simulink model "PlatooningUsingV2VTestBench"  (R2025a)
settings: Solver=ode23tb  StartTime=0.0  StopTime=stopTime  RelTol=1e-1  AbsTol=5e-5
PostLoadFcn:
  | helperSLPlatooningUsingV2VSetup
InitFcn:
  | figureName = 'Platooning Simulation Results';
  | hFig = findobj('Type','Figure','Name',figureName);
  | close(hFig)
values from neighbouring files (symbols this model uses):
  L = vehicleDimension.TractorLength + vehicleDimension.TrailerLength + vehicleDimension.InterConnection - vehicleDimension.Overlap + spacing    [helperSLPlatooningUsingV2VSetup.m]
  spacing = 7    [helperSLPlatooningUsingV2VSetup.m]
undefined symbols (not defined in the file or in its folder): accelerationProfile, C1, DiscIntNeverNeededParam, initialActorPose, K1, K2, N, sceneOrigin, Sim3dSensor, tractor, Ts, Tsv, vehicleDimension
libraries: simulink x7, sim3dautolib x6, slpidlib x2, sim3dcameralib x1, sim3dlib x1, visionsinks x1
(part 2 of 2)

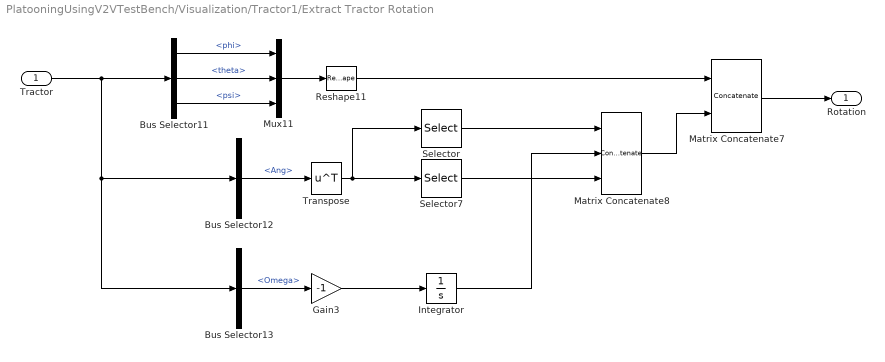
== system PlatooningUsingV2VTestBench/Visualization/Tractor1/Extract Tractor Rotation ==
  Tractor : Inport
  Bus Selector11 : BusSelector  OutputSignals=Vehicle.InertFrm.Cg.Ang.phi,Vehicle.InertFrm.Cg.Ang.theta,Vehicle.InertFrm.Cg.Ang.psi
  Bus Selector12 : BusSelector  OutputSignals=Suspension.Whl.Ang
  Bus Selector13 : BusSelector  OutputSignals=Wheels.TireFrame.Omega
  Gain3 : Gain  Gain=-1
  Integrator : Integrator
  Matrix Concatenate7 : Concatenate  Mode=Multidimensional array
  Matrix Concatenate8 : Concatenate  NumInputs=3  Mode=Multidimensional array  ConcatenateDimension=2
  Mux11 : Mux  Inputs=3
  Reshape11 : Reshape  OutputDimensionality=Row vector (2-D)
  Selector : Selector  NumberOfDimensions=2  InputPortWidth=3  IndexOptions=Select all,Index vector (dialog)  Indices=1,1  OutputSizes=1,1
  Selector7 : Selector  NumberOfDimensions=2  InputPortWidth=3  IndexOptions=Select all,Index vector (dialog)  Indices=3,3  OutputSizes=1,1
  Transpose : Math  Operator=transpose
  Rotation : Outport
  wires:
  Transpose/1 -> Selector7/1, Selector/1
  Gain3/1 -> Integrator/1
  Selector7/1 -> Matrix Concatenate8/3
  Bus Selector11/3 -> Mux11/3  "<psi>"
  Bus Selector11/1 -> Mux11/1  "<phi>"
  Bus Selector11/2 -> Mux11/2  "<theta>"
  Reshape11/1 -> Matrix Concatenate7/1
  Selector/1 -> Matrix Concatenate8/1
  Mux11/1 -> Reshape11/1
  Bus Selector12/1 -> Transpose/1  "<Ang>"
  Matrix Concatenate8/1 -> Matrix Concatenate7/2
  Tractor/1 -> Bus Selector13/1, Bus Selector12/1, Bus Selector11/1
  Bus Selector13/1 -> Gain3/1  "<Omega>"
  Integrator/1 -> Matrix Concatenate8/2
  Matrix Concatenate7/1 -> Rotation/1

== system PlatooningUsingV2VTestBench/Visualization/Tractor1/Extract Tractor Translation ==
  Tractor : Inport
  Bus Selector3 : BusSelector  OutputSignals=Wheels.TireFrame.z
  Bus Selector8 : BusSelector  OutputSignals=Vehicle.InertFrm.Hitch.Disp.X,Vehicle.InertFrm.Hitch.Disp.Y,Vehicle.InertFrm.Hitch.Disp.Z
  Constant : Constant  Value=tractor.HeightCG-tractor.HitchHeight
  Constant1 : Constant  Value=zeros(6,2)
  Matrix Concatenate1 : Concatenate  Mode=Multidimensional array  ConcatenateDimension=2
  Matrix Concatenate5 : Concatenate  Mode=Multidimensional array
  Mux8 : Mux  Inputs=3
  Reshape : Reshape  OutputDimensionality=Column vector (2-D)
  Reshape8 : Reshape  OutputDimensionality=Row vector (2-D)
  Sum : Sum  Inputs=|+-
  Translation : Outport
  wires:
  Reshape8/1 -> Matrix Concatenate5/1
  Bus Selector8/3 -> Sum/1  "<Z>"
  Sum/1 -> Mux8/3
  Bus Selector8/1 -> Mux8/1  "<X>"
  Constant/1 -> Sum/2
  Mux8/1 -> Reshape8/1
  Matrix Concatenate5/1 -> Translation/1
  Bus Selector8/2 -> Mux8/2  "<Y>"
  Tractor/1 -> Bus Selector8/1, Bus Selector3/1
  Bus Selector3/1 -> Reshape/1  "<z>"
  Reshape/1 -> Matrix Concatenate1/2
  Constant1/1 -> Matrix Concatenate1/1
  Matrix Concatenate1/1 -> Matrix Concatenate5/2

== system PlatooningUsingV2VTestBench/Visualization/Trailer/Extract Trailer Rotation ==
  Trailer : Inport
  Bus Selector11 : BusSelector  OutputSignals=Vehicle.InertFrm.Cg.Ang.phi,Vehicle.InertFrm.Cg.Ang.theta,Vehicle.InertFrm.Cg.Ang.psi
  Bus Selector12 : BusSelector  OutputSignals=Suspension.Whl.Ang
  Bus Selector13 : BusSelector  OutputSignals=Wheels.TireFrame.Omega
  Gain3 : Gain  Gain=-1
  Integrator : Integrator
  Matrix Concatenate7 : Concatenate  Mode=Multidimensional array
  Matrix Concatenate8 : Concatenate  NumInputs=3  Mode=Multidimensional array  ConcatenateDimension=2
  Mux11 : Mux  Inputs=3
  Reshape11 : Reshape  OutputDimensionality=Row vector (2-D)
  Selector : Selector  NumberOfDimensions=2  InputPortWidth=3  IndexOptions=Select all,Index vector (dialog)  Indices=1,1  OutputSizes=1,1
  Selector7 : Selector  NumberOfDimensions=2  InputPortWidth=3  IndexOptions=Select all,Index vector (dialog)  Indices=3,3  OutputSizes=1,1
  Transpose : Math  Operator=transpose
  Rotation : Outport
  wires:
  Matrix Concatenate7/1 -> Rotation/1
  Integrator/1 -> Matrix Concatenate8/2
  Bus Selector13/1 -> Gain3/1  "<Omega>"
  Trailer/1 -> Bus Selector11/1, Bus Selector12/1, Bus Selector13/1
  Matrix Concatenate8/1 -> Matrix Concatenate7/2
  Bus Selector12/1 -> Transpose/1  "<Ang>"
  Mux11/1 -> Reshape11/1
  Selector/1 -> Matrix Concatenate8/1
  Reshape11/1 -> Matrix Concatenate7/1
  Bus Selector11/2 -> Mux11/2  "<theta>"
  Bus Selector11/1 -> Mux11/1  "<phi>"
  Bus Selector11/3 -> Mux11/3  "<psi>"
  Selector7/1 -> Matrix Concatenate8/3
  Gain3/1 -> Integrator/1
  Transpose/1 -> Selector/1, Selector7/1

== system PlatooningUsingV2VTestBench/Visualization/Trailer/Extract Trailer Translation ==
  Trailer : Inport
  Bus Selector3 : BusSelector  OutputSignals=Wheels.TireFrame.z
  Bus Selector8 : BusSelector  OutputSignals=Vehicle.InertFrm.HitchF.Disp.X,Vehicle.InertFrm.HitchF.Disp.Y,Vehicle.InertFrm.HitchF.Disp.Z
  Constant : Constant  Value=trailer.HeightCG-trailer.HitchHeight
  Constant1 : Constant  Value=zeros(6,2)
  Matrix Concatenate1 : Concatenate  Mode=Multidimensional array  ConcatenateDimension=2
  Matrix Concatenate5 : Concatenate  Mode=Multidimensional array
  Mux8 : Mux  Inputs=3
  Reshape : Reshape  OutputDimensionality=Column vector (2-D)
  Reshape8 : Reshape  OutputDimensionality=Row vector (2-D)
  Sum : Sum  Inputs=|+-
  Translation : Outport
  wires:
  Bus Selector8/3 -> Sum/1  "<Z>"
  Matrix Concatenate5/1 -> Translation/1
  Constant/1 -> Sum/2
  Trailer/1 -> Bus Selector3/1, Bus Selector8/1
  Bus Selector8/2 -> Mux8/2  "<Y>"
  Bus Selector3/1 -> Reshape/1  "<z>"
  Matrix Concatenate1/1 -> Matrix Concatenate5/2
  Reshape8/1 -> Matrix Concatenate5/1
  Mux8/1 -> Reshape8/1
  Reshape/1 -> Matrix Concatenate1/2
  Sum/1 -> Mux8/3
  Constant1/1 -> Matrix Concatenate1/1
  Bus Selector8/1 -> Mux8/1  "<X>"

== system PlatooningUsingV2VTestBench/Visualization/Trailer1/Extract Trailer Rotation ==
  Trailer : Inport
  Bus Selector11 : BusSelector  OutputSignals=Vehicle.InertFrm.Cg.Ang.phi,Vehicle.InertFrm.Cg.Ang.theta,Vehicle.InertFrm.Cg.Ang.psi
  Bus Selector12 : BusSelector  OutputSignals=Suspension.Whl.Ang
  Bus Selector13 : BusSelector  OutputSignals=Wheels.TireFrame.Omega
  Gain3 : Gain  Gain=-1
  Integrator : Integrator
  Matrix Concatenate7 : Concatenate  Mode=Multidimensional array
  Matrix Concatenate8 : Concatenate  NumInputs=3  Mode=Multidimensional array  ConcatenateDimension=2
  Mux11 : Mux  Inputs=3
  Reshape11 : Reshape  OutputDimensionality=Row vector (2-D)
  Selector : Selector  NumberOfDimensions=2  InputPortWidth=3  IndexOptions=Select all,Index vector (dialog)  Indices=1,1  OutputSizes=1,1
  Selector7 : Selector  NumberOfDimensions=2  InputPortWidth=3  IndexOptions=Select all,Index vector (dialog)  Indices=3,3  OutputSizes=1,1
  Transpose : Math  Operator=transpose
  Rotation : Outport
  wires:
  Matrix Concatenate7/1 -> Rotation/1
  Integrator/1 -> Matrix Concatenate8/2
  Bus Selector13/1 -> Gain3/1  "<Omega>"
  Trailer/1 -> Bus Selector11/1, Bus Selector12/1, Bus Selector13/1
  Matrix Concatenate8/1 -> Matrix Concatenate7/2
  Bus Selector12/1 -> Transpose/1  "<Ang>"
  Mux11/1 -> Reshape11/1
  Selector/1 -> Matrix Concatenate8/1
  Reshape11/1 -> Matrix Concatenate7/1
  Bus Selector11/2 -> Mux11/2  "<theta>"
  Bus Selector11/1 -> Mux11/1  "<phi>"
  Bus Selector11/3 -> Mux11/3  "<psi>"
  Selector7/1 -> Matrix Concatenate8/3
  Gain3/1 -> Integrator/1
  Transpose/1 -> Selector/1, Selector7/1

== system PlatooningUsingV2VTestBench/Visualization/Trailer1/Extract Trailer Translation ==
  Trailer : Inport
  Bus Selector3 : BusSelector  OutputSignals=Wheels.TireFrame.z
  Bus Selector8 : BusSelector  OutputSignals=Vehicle.InertFrm.HitchF.Disp.X,Vehicle.InertFrm.HitchF.Disp.Y,Vehicle.InertFrm.HitchF.Disp.Z
  Constant : Constant  Value=trailer.HeightCG-trailer.HitchHeight
  Constant1 : Constant  Value=zeros(6,2)
  Matrix Concatenate1 : Concatenate  Mode=Multidimensional array  ConcatenateDimension=2
  Matrix Concatenate5 : Concatenate  Mode=Multidimensional array
  Mux8 : Mux  Inputs=3
  Reshape : Reshape  OutputDimensionality=Column vector (2-D)
  Reshape8 : Reshape  OutputDimensionality=Row vector (2-D)
  Sum : Sum  Inputs=|+-
  Translation : Outport
  wires:
  Bus Selector8/3 -> Sum/1  "<Z>"
  Matrix Concatenate5/1 -> Translation/1
  Constant/1 -> Sum/2
  Trailer/1 -> Bus Selector3/1, Bus Selector8/1
  Bus Selector8/2 -> Mux8/2  "<Y>"
  Bus Selector3/1 -> Reshape/1  "<z>"
  Matrix Concatenate1/1 -> Matrix Concatenate5/2
  Reshape8/1 -> Matrix Concatenate5/1
  Mux8/1 -> Reshape8/1
  Reshape/1 -> Matrix Concatenate1/2
  Sum/1 -> Mux8/3
  Constant1/1 -> Matrix Concatenate1/1
  Bus Selector8/1 -> Mux8/1  "<X>"

== matlab function PlatooningUsingV2VTestBench/Pack BSM/MATLAB Function ==
  data: u input; y output
function y = computeNumOfBSM(u)
    y = 0;
    y = size(u,1);
end

== matlab function PlatooningUsingV2VTestBench/Follower1/findLeadAndFrontVehicles ==
  data: leadAndFrontInfo output Bus: BusLeadAndFrontInfo; bsm input Bus: BusBSM; leaderAcceleration output; leaderVelocity output; frontAcceleration output; frontPosition output; origin input; egoID parameter; egoPosition input; outputStruct parameter
function [leadAndFrontInfo, leaderAcceleration, leaderVelocity, frontAcceleration, frontPosition] = findLeadAndFrontVehicles(bsm,origin,egoID,egoPosition, outputStruct)
% Initialize output
leaderAcceleration = 0;
leaderVelocity = 0;
frontAcceleration = 0;
frontPosition = 0;
leadAndFrontInfo = outputStruct; 
% Read the pose information from bsm
[position, velocity, acceleration] = readPose(bsm,origin,egoID);
% Sort the position to find lead and front
[key,index] = sort(position(:,1)-egoPosition(:,1),'descend');
% Find lead and front
if ~isempty(key) && key(1)>0
    leadIdx = index(1);
    leaderVelocity = velocity(leadIdx);
    leaderAcceleration = acceleration(leadIdx);
    sz = size(key,1);
    frontIdx = 0;
    frontVelocity = 0;
    for j = 1:sz
        if key(j) < 0
            frontIdx = index(j-1);
            frontPosition     = position(frontIdx,1);
            frontVelocity     = velocity(frontIdx);
            frontAcceleration = acceleration(frontIdx); 
            break;
        end
    end
    % Fill the Lead and Front data from BSM into the output struct
    leadAndFrontInfo.NumOfReceivedBSM = bsm.NumOfBSM-1; % Remove Self
    leadAndFrontInfo.ID = egoID;
    leadAndFrontInfo.LeadPosition  = position(leadIdx,:);
    leadAndFrontInfo.LeadSpeed     = leaderVelocity;
    leadAndFrontInfo.FrontPosition = position(frontIdx,:);
    leadAndFrontInfo.FrontSpeed    = frontVelocity;
end
end

function [pos, vel, acc] = readPose(bsm,origin,egoID)
    pos = zeros(bsm.NumOfBSM,3);
    vel = zeros(bsm.NumOfBSM,1);
    acc = zeros(bsm.NumOfBSM,1);
    for i = 1:bsm.NumOfBSM
        if bsm.BSMCoreData(i).Id ~= egoID
            % Convert to double
            lla = [double(bsm.BSMCoreData(i).Lattitude)*10^-7,double(bsm.BSMCoreData(i).Longitude)*10^-7,double(bsm.BSMCoreData(i).Elevation)*0.1];
            % Transform geodetic coordinates to local east-north-up coordinates
            x = 0;
            y = 0;
            z = 0;
            [x,y,z] = latlon2local(lla(1),lla(2),lla(3),origin);
            % add to the output
            pos(i,:) = [x y z];
            vel(i) = double(bsm.BSMCoreData(i).Speed)*0.02;
            acc(i) = double(bsm.BSMCoreData(i).AccelSet.LongAcc)*0.01;
        else
            pos(i,:) = [-inf -inf -inf];
            vel(i) = -inf;
            acc(i) = -inf;
        end
    end
end

== matlab function PlatooningUsingV2VTestBench/Follower2/findLeadAndFrontVehicles ==
  data: leadAndFrontInfo output Bus: BusLeadAndFrontInfo; bsm input Bus: BusBSM; leaderAcceleration output; leaderVelocity output; frontAcceleration output; frontPosition output; origin input; egoID parameter; egoPosition input; outputStruct parameter
function [leadAndFrontInfo, leaderAcceleration, leaderVelocity, frontAcceleration, frontPosition] = findLeadAndFrontVehicles(bsm,origin,egoID,egoPosition, outputStruct)
% Initialize output
leaderAcceleration = 0;
leaderVelocity = 0;
frontAcceleration = 0;
frontPosition = 0;
leadAndFrontInfo = outputStruct; 
% Read the pose information from bsm
[position, velocity, acceleration] = readPose(bsm,origin,egoID);
% Sort the position to find lead and front
[key,index] = sort(position(:,1)-egoPosition(:,1),'descend');
% Find lead and front
if ~isempty(key) && key(1)>0
    leadIdx = index(1);
    leaderVelocity = velocity(leadIdx);
    leaderAcceleration = acceleration(leadIdx);
    sz = size(key,1);
    frontIdx = 0;
    frontVelocity = 0;
    for j = 1:sz
        if key(j) < 0
            frontIdx = index(j-1);
            frontPosition     = position(frontIdx,1);
            frontVelocity     = velocity(frontIdx);
            frontAcceleration = acceleration(frontIdx); 
            break;
        end
    end
    % Fill the Lead and Front data from BSM into the output struct
    leadAndFrontInfo.NumOfReceivedBSM = bsm.NumOfBSM-1;
    leadAndFrontInfo.ID = egoID;
    leadAndFrontInfo.LeadPosition  = position(leadIdx,:);
    leadAndFrontInfo.LeadSpeed     = leaderVelocity;
    leadAndFrontInfo.FrontPosition = position(frontIdx,:);
    leadAndFrontInfo.FrontSpeed    = frontVelocity;
end
end

function [pos, vel, acc] = readPose(bsm,origin,egoID)
    pos = zeros(bsm.NumOfBSM,3);
    vel = zeros(bsm.NumOfBSM,1);
    acc = zeros(bsm.NumOfBSM,1);
    for i = 1:bsm.NumOfBSM
        if bsm.BSMCoreData(i).Id ~= egoID
            % Convert to double
            lla = [double(bsm.BSMCoreData(i).Lattitude)*10^-7,double(bsm.BSMCoreData(i).Longitude)*10^-7,double(bsm.BSMCoreData(i).Elevation)*0.1];
            % Transform geodetic coordinates to local east-north-up coordinates
            x = 0;
            y = 0;
            z = 0;
            [x,y,z] = latlon2local(lla(1),lla(2),lla(3),origin);
            % add to the output
            pos(i,:) = [x y z];
            vel(i) = double(bsm.BSMCoreData(i).Speed)*0.02;
            acc(i) = double(bsm.BSMCoreData(i).AccelSet.LongAcc)*0.01;
        else
            pos(i,:) = [-inf -inf -inf];
            vel(i) = -inf;
            acc(i) = -inf;
        end
    end
end

== matlab function PlatooningUsingV2VTestBench/Metrics/Compute Spacing ==
  data: isPlatoonFormed output; leader input; follower1 input; follower2 input; spacing12 output; spacing23 output; expectedSpacing parameter
function [isPlatoonFormed,spacing12,spacing23] = computeSpacing(leader,follower1,follower2,expectedSpacing)
    persistent platoonFormed
    if isempty(platoonFormed)
        platoonFormed = false;
    end
    % Spacing Between Leader and Follower 1
    spacing12 = leader.Actors.Position(1) - follower1.Actors.Position(1);
    % Spacing Between Follower 1 and Follower 2
    spacing23 = follower1.Actors.Position(1) - follower2.Actors.Position(1);
    % Check is platoon is formed
    spacingTolerance = 5;
    if ~platoonFormed && abs(expectedSpacing - spacing12)<=spacingTolerance && abs(expectedSpacing - spacing23)<=spacingTolerance
        platoonFormed = true;
    end
    isPlatoonFormed = platoonFormed;
end

== matlab function PlatooningUsingV2VTestBench/Visualization/Extract Translation and Rotation /Get Rotation ==
  data: rotation output; angularPos input
function rotation = fcn(angularPos)
    y = repmat(angularPos,6,1);
    rotation = [0 0 0;zeros(6,1) y zeros(6,1)];
end

== matlab function PlatooningUsingV2VTestBench/Follower1/Pack Actor Info ==
  data: acceleration input; position input; velocity input; actorInfo output Bus: BusActorsInfo; outputStruct parameter; initialActorInfo parameter; time input
function actorInfo = packActorInfo(acceleration,position,velocity,outputStruct,initialActorInfo,time)

actorInfo = outputStruct;
actorInfo.NumActors = 1;
actorInfo.Time = time;
actorInfo.Actors.ActorID      = initialActorInfo.ActorID;
actorInfo.Actors.ClassID      = initialActorInfo.ClassID;
actorInfo.Actors.Position     = [position(1) position(2) position(3)];
actorInfo.Actors.Velocity     = [velocity(1) velocity(2) velocity(3)];
actorInfo.Actors.Acceleration = [acceleration(1) acceleration(2) acceleration(3)];
actorInfo.Actors.Length       = initialActorInfo.Length;
actorInfo.Actors.Width        = initialActorInfo.Width;
end

== matlab function PlatooningUsingV2VTestBench/Follower2/Pack Actor Info ==
  data: acceleration input; position input; velocity input; actorInfo output Bus: BusActorsInfo; outputStruct parameter; initialActorInfo parameter; time input
function actorInfo = packActorInfo(acceleration,position,velocity,outputStruct,initialActorInfo,time)

actorInfo = outputStruct;
actorInfo.NumActors = 1;
actorInfo.Time = time;
actorInfo.Actors.ActorID      = initialActorInfo.ActorID;
actorInfo.Actors.ClassID      = initialActorInfo.ClassID;
actorInfo.Actors.Position     = [position(1) position(2) position(3)];
actorInfo.Actors.Velocity     = [velocity(1) velocity(2) velocity(3)];
actorInfo.Actors.Acceleration = [acceleration(1) acceleration(2) acceleration(3)];
actorInfo.Actors.Length       = initialActorInfo.Length;
actorInfo.Actors.Width        = initialActorInfo.Width;
end

== matlab function PlatooningUsingV2VTestBench/Leader/Pack Actor Info ==
  data: acceleration input; velocity input; position input; actorInfo output Bus: BusActorsInfo; outputStruct parameter; initialActorInfo parameter; time input
function actorInfo = packActorInfo(acceleration,velocity,position,outputStruct,initialActorInfo,time)

actorInfo = outputStruct;
actorInfo.NumActors = 1;
actorInfo.Time = time;
actorInfo.Actors.ActorID      = initialActorInfo.ActorID;
actorInfo.Actors.ClassID      = initialActorInfo.ClassID;
actorInfo.Actors.Position     = [position(1) position(2) 0];
actorInfo.Actors.Velocity     = [velocity(1) velocity(2) 0];
actorInfo.Actors.Acceleration = [acceleration(1) acceleration(2) 0];
actorInfo.Actors.Length       = initialActorInfo.Length;
actorInfo.Actors.Width        = initialActorInfo.Width;
end
